simulink model "PreCNN_SAC_RL_env"  (R2025b)
settings: Solver=ode4  StartTime=0.0  StopTime=50  FixedStep=0.005  RelTol=1e-3  EnableMultiTasking=on
values from neighbouring files (symbols this model uses):
  dyn_obs = struct('p0', cell(1, num_dyn_obs), 'v', cell(1, num_dyn_obs), 'radius', cell(1, num_dyn_obs))    [genera_ostacoli_dinamici.m]    (also in visualizza_raggi_completo.m = scenario.dynamic_obstacles)
  initialGainsMultiplier = 15    [init_rl.m]    (also in report_agent.m; test.m; test_agent.m; train.m)
  logging = true    [train.m]    (also in train_agent.m; train_agent_precedente.m)
  Ts = 0.1    [init_rl.m]    (also in report_agent.m; test.m; test_agent.m; train.m)
undefined symbols (not defined in the file or in its folder): angControlTuning, angRateControlTuning, bounds, Controller, decyear, DiscIntNeverNeededParam, DroneMass, Dz, Gravity, initialConditions, Iz, leapyear, logPath_num, Nz, posControlTuning, Pz, startFlightTime, tunePositionController, UAVSampleTime, Vehicle, velControlTuning
libraries: slpidlib x14, slctrl_autotuning x8, sharedutil x4, aerolibconvert2 x3, aerolibatmos2 x2, aerolibgravity2 x2, shared6dof x2, aerolibasang x2, sensorinslib x2, deeplib x1, rllib x1, matrix_library x1
(part 4 of 5)

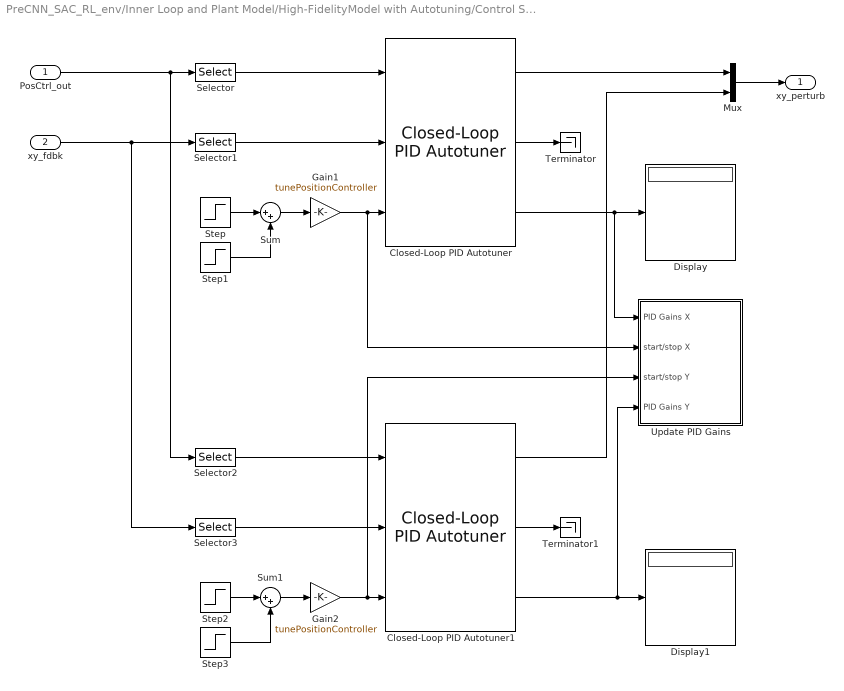
== system PreCNN_SAC_RL_env/Inner Loop and Plant Model/High-FidelityModel with Autotuning/Control System/Controller/Position Controller/Position Loop Autotuning ==
  PosCtrl_out : Inport
  xy_fdbk : Inport  Port=2
  Closed-Loop PID Autotuner : slctrl_autotuning/Closed-Loop PID Autotuner  PIDType=P  PIDForm=Parallel  TimeDomain=discrete-time  DiscreteTs=UAVSampleTime  TuningTs=0.2  UseTuningTs=off  IntegratorFormula=Forward Euler  FilterFormula=Forward Euler  ContinuousTs=0.02  Bandwidth=posControlTuning.wc  UseExternalWC=off  TargetPM=posControlTuning.pm  UseExternalPM=off  UseExternalAchievedPM=off  ExperimentMode=Superposition  PlantType=Stable  PlantSign=Positive  AmpSine=posControlTuning.sineAmp  UseExternalAmpSine=off  UseExternalFRD=off  UseExternalU0=off  UseCompanion=off  NotDeployTuningModule=off  UsePLCCoder=off  OutputMode=perturbation only  BlockDataType=single  UseExperimentGoodPort=off  UseConnectedPID=on  blockpath=[]  tunedP=0  tunedI=0  tunedD=0  tunedN=100  tunedPM=0  EstimationWindowSize=3  UseExternalTuningParams=off  SingleMultiRateVariant=SingleSamplingRate  NumEstimationPeriods=4  NumSettlingPeriods=2  NumOfPRBSPeriod=1  PRBSSignalOrder=12  ExperimentModeVariant=VariantSuperimposed  OutputChoice=VariantDonly  ConvergenceCalcVariant=ConvSuperpositionPRBSVariant
  Closed-Loop PID Autotuner1 : slctrl_autotuning/Closed-Loop PID Autotuner  PIDType=P  PIDForm=Parallel  TimeDomain=discrete-time  DiscreteTs=UAVSampleTime  TuningTs=0.2  UseTuningTs=off  IntegratorFormula=Forward Euler  FilterFormula=Forward Euler  ContinuousTs=0.02  Bandwidth=posControlTuning.wc  UseExternalWC=off  TargetPM=posControlTuning.pm  UseExternalPM=off  UseExternalAchievedPM=off  ExperimentMode=Superposition  PlantType=Stable  PlantSign=Positive  AmpSine=posControlTuning.sineAmp  UseExternalAmpSine=off  UseExternalFRD=off  UseExternalU0=off  UseCompanion=off  NotDeployTuningModule=off  UsePLCCoder=off  OutputMode=perturbation only  BlockDataType=single  UseExperimentGoodPort=off  UseConnectedPID=on  blockpath=[]  tunedP=0  tunedI=0  tunedD=0  tunedN=100  tunedPM=0  EstimationWindowSize=3  UseExternalTuningParams=off  SingleMultiRateVariant=SingleSamplingRate  NumEstimationPeriods=4  NumSettlingPeriods=2  NumOfPRBSPeriod=1  PRBSSignalOrder=12  ExperimentModeVariant=VariantSuperimposed  OutputChoice=VariantDonly  ConvergenceCalcVariant=ConvSuperpositionPRBSVariant
  Display : Display
  Display1 : Display
  Gain1 : Gain  Gain=tunePositionController
  Gain2 : Gain  Gain=tunePositionController
  Mux : Mux  Inputs=2
  Selector : Selector  InputPortWidth=2  IndexOptions=Index vector (dialog)  Indices=1  OutputSizes=1
  Selector1 : Selector  InputPortWidth=2  IndexOptions=Index vector (dialog)  Indices=1  OutputSizes=1
  Selector2 : Selector  InputPortWidth=2  IndexOptions=Index vector (dialog)  Indices=2  OutputSizes=1
  Selector3 : Selector  InputPortWidth=2  IndexOptions=Index vector (dialog)  Indices=2  OutputSizes=1
  Step : Step  Time=posControlTuning.startExpX  SampleTime=UAVSampleTime
  Step1 : Step  Time=posControlTuning.stopExpX  After=-1  SampleTime=UAVSampleTime
  Step2 : Step  Time=posControlTuning.startExpY  SampleTime=UAVSampleTime
  Step3 : Step  Time=posControlTuning.stopExpY  After=-1  SampleTime=UAVSampleTime
  Sum : Sum  Inputs=|++
  Sum1 : Sum  Inputs=|++
  Terminator : Terminator
  Terminator1 : Terminator
  Update PID Gains : Subsystem
  xy_perturb : Outport
  wires:
  PosCtrl_out/1 -> Selector2/1, Selector/1
  xy_fdbk/1 -> Selector3/1, Selector1/1
  Selector/1 -> Closed-Loop PID Autotuner/1
  Selector1/1 -> Closed-Loop PID Autotuner/2
  Sum/1 -> Gain1/1
  Step/1 -> Sum/1
  Step1/1 -> Sum/2
  Closed-Loop PID Autotuner/2 -> Terminator/1
  Mux/1 -> xy_perturb/1
  Closed-Loop PID Autotuner/1 -> Mux/1
  Selector2/1 -> Closed-Loop PID Autotuner1/1
  Selector3/1 -> Closed-Loop PID Autotuner1/2
  Step3/1 -> Sum1/2
  Step2/1 -> Sum1/1
  Sum1/1 -> Gain2/1
  Closed-Loop PID Autotuner1/2 -> Terminator1/1
  Closed-Loop PID Autotuner1/1 -> Mux/2
  Closed-Loop PID Autotuner/3 -> Update PID Gains/1(PID Gains X), Display/1
  Closed-Loop PID Autotuner1/3 -> Update PID Gains/4(PID Gains Y), Display1/1
  Gain1/1 -> Update PID Gains/2(start/stop X), Closed-Loop PID Autotuner/3
  Gain2/1 -> Update PID Gains/3(start/stop Y), Closed-Loop PID Autotuner1/3

== system PreCNN_SAC_RL_env/Inner Loop and Plant Model/High-FidelityModel with Autotuning/Control System/Controller/Position Controller/Velocity Loop Autotuning ==
  VelCtrl_out : Inport
  xxyy_fdbk : Inport  Port=2
  Closed-Loop PID Autotuner : slctrl_autotuning/Closed-Loop PID Autotuner  PIDType=PI  PIDForm=Parallel  TimeDomain=discrete-time  DiscreteTs=UAVSampleTime  TuningTs=0.2  UseTuningTs=off  IntegratorFormula=Forward Euler  FilterFormula=Forward Euler  ContinuousTs=0.02  Bandwidth=velControlTuning.wc  UseExternalWC=off  TargetPM=velControlTuning.pm  UseExternalPM=off  UseExternalAchievedPM=off  ExperimentMode=Superposition  PlantType=Stable  PlantSign=Positive  AmpSine=velControlTuning.sineAmp  UseExternalAmpSine=off  UseExternalFRD=off  UseExternalU0=off  UseCompanion=off  NotDeployTuningModule=off  UsePLCCoder=off  OutputMode=perturbation only  BlockDataType=single  UseExperimentGoodPort=off  UseConnectedPID=on  blockpath=[]  tunedP=0  tunedI=0  tunedD=0  tunedN=100  tunedPM=0  EstimationWindowSize=3  UseExternalTuningParams=off  SingleMultiRateVariant=SingleSamplingRate  NumEstimationPeriods=4  NumSettlingPeriods=2  NumOfPRBSPeriod=1  PRBSSignalOrder=12  ExperimentModeVariant=VariantSuperimposed  OutputChoice=VariantDonly  ConvergenceCalcVariant=ConvSuperpositionPRBSVariant
  Closed-Loop PID Autotuner1 : slctrl_autotuning/Closed-Loop PID Autotuner  PIDType=PI  PIDForm=Parallel  TimeDomain=discrete-time  DiscreteTs=UAVSampleTime  TuningTs=0.2  UseTuningTs=off  IntegratorFormula=Forward Euler  FilterFormula=Forward Euler  ContinuousTs=0.02  Bandwidth=velControlTuning.wc  UseExternalWC=off  TargetPM=velControlTuning.pm  UseExternalPM=off  UseExternalAchievedPM=off  ExperimentMode=Superposition  PlantType=Stable  PlantSign=Positive  AmpSine=velControlTuning.sineAmp  UseExternalAmpSine=off  UseExternalFRD=off  UseExternalU0=off  UseCompanion=off  NotDeployTuningModule=off  UsePLCCoder=off  OutputMode=perturbation only  BlockDataType=single  UseExperimentGoodPort=off  UseConnectedPID=on  blockpath=[]  tunedP=0  tunedI=0  tunedD=0  tunedN=100  tunedPM=0  EstimationWindowSize=3  UseExternalTuningParams=off  SingleMultiRateVariant=SingleSamplingRate  NumEstimationPeriods=4  NumSettlingPeriods=2  NumOfPRBSPeriod=1  PRBSSignalOrder=12  ExperimentModeVariant=VariantSuperimposed  OutputChoice=VariantDonly  ConvergenceCalcVariant=ConvSuperpositionPRBSVariant
  Display : Display
  Display1 : Display
  Gain : Gain  Gain=tunePositionController
  Gain1 : Gain  Gain=tunePositionController
  Mux : Mux  Inputs=2
  Scope : Scope
      settings: ActiveDisplayYMinimum=99.18257  ActiveDisplayYMaximum=100.62707  DataLoggingVariableName=ScopeData9
  Scope1 : Scope
      settings: DataLoggingVariableName=ScopeData10
  Selector : Selector  InputPortWidth=2  IndexOptions=Index vector (dialog)  Indices=1  OutputSizes=1
  Selector1 : Selector  InputPortWidth=2  IndexOptions=Index vector (dialog)  Indices=1  OutputSizes=1
  Selector2 : Selector  InputPortWidth=2  IndexOptions=Index vector (dialog)  Indices=2  OutputSizes=1
  Selector3 : Selector  InputPortWidth=2  IndexOptions=Index vector (dialog)  Indices=2  OutputSizes=1
  Step : Step  Time=velControlTuning.startExpX  SampleTime=UAVSampleTime
  Step1 : Step  Time=velControlTuning.stopExpX  After=-1  SampleTime=UAVSampleTime
  Step2 : Step  Time=velControlTuning.startExpY  SampleTime=UAVSampleTime
  Step3 : Step  Time=velControlTuning.stopExpY  After=-1  SampleTime=UAVSampleTime
  Sum : Sum  Inputs=|++
  Sum1 : Sum  Inputs=|++
  Update PID Gains : Subsystem
  xxyy_perturb : Outport
  wires:
  Closed-Loop PID Autotuner1/1 -> Mux/2
  Closed-Loop PID Autotuner1/2 -> Scope1/1
  Sum1/1 -> Gain1/1
  Step2/1 -> Sum1/1
  Step3/1 -> Sum1/2
  Selector3/1 -> Closed-Loop PID Autotuner1/2
  Selector2/1 -> Closed-Loop PID Autotuner1/1
  Closed-Loop PID Autotuner/1 -> Mux/1
  Mux/1 -> xxyy_perturb/1
  Closed-Loop PID Autotuner/2 -> Scope/1
  Step1/1 -> Sum/2
  Step/1 -> Sum/1
  Sum/1 -> Gain/1
  Selector1/1 -> Closed-Loop PID Autotuner/2
  Selector/1 -> Closed-Loop PID Autotuner/1
  xxyy_fdbk/1 -> Selector1/1, Selector3/1
  VelCtrl_out/1 -> Selector/1, Selector2/1
  Closed-Loop PID Autotuner/3 -> Update PID Gains/1(PID Gains XX), Display/1
  Closed-Loop PID Autotuner1/3 -> Update PID Gains/4(PID Gains YY), Display1/1
  Gain/1 -> Update PID Gains/2(start/stop XX), Closed-Loop PID Autotuner/3
  Gain1/1 -> Update PID Gains/3(start/stop YY), Closed-Loop PID Autotuner1/3

== system PreCNN_SAC_RL_env/Inner Loop and Plant Model/High-FidelityModel with Autotuning/Plant Model/AC model/Drag Calculation/Drag Calc ==
  Density : Inport  Unit=kg/m^3
  vel : Inport  Port=2  Unit=m/s
  Dynamic Pressure : aerolibasang/Dynamic Pressure
  Gain : Gain  Gain=[.25 .25]
  Mux1 : Mux  Inputs=2
  Product : Product  Inputs=3  RndMeth=Zero
  diameter : Constant  Value=Vehicle.Airframe.diameter  SampleTime=0
  dragCoeff : Constant  Value=Vehicle.Airframe.Cdx  SampleTime=0
  drag : Outport  Unit=N  VectorParamsAs1DForOutWhenUnconnected=off
  wires:
  Product/1 -> drag/1
  dragCoeff/1 -> Product/3  "Cd"
  Dynamic Pressure/1 -> Product/1  "q"
  diameter/1 -> Gain/1, Mux1/2
  Mux1/1 -> Product/2  "S"
  Gain/1 -> Mux1/1
  vel/1 -> Dynamic Pressure/1
  Density/1 -> Dynamic Pressure/2

== system PreCNN_SAC_RL_env/Inner Loop and Plant Model/High-FidelityModel with Autotuning/Plant Model/AC model/Motor Forces and Torques/For Each Subsystem ==
  Vb : Inport  PortDimensions=3
  rho : Inport  Port=2  PortDimensions=1
  Omega : Inport  Port=3
  w : Inport  Port=4  Partition=on  PartitionDimension=2  PartitionWidth=1  PartitionOffset=0
  D : Inport  Port=5  Partition=on  PartitionDimension=2  PartitionWidth=1  PartitionOffset=0
  For Each : ForEach  DisableCoverage=on
  RotorDynamics : Subsystem  TreatAsAtomicUnit=on
      mask init:
      | aeroicon('aeroblk');
      settings: RTWFcnNameOpts=Use subsystem name  RTWFileNameOpts=Use function name
  Forces : Outport  ConcatenationDimension=2  VectorParamsAs1DForOutWhenUnconnected=off
  Moments : Outport  Port=2  ConcatenationDimension=2  VectorParamsAs1DForOutWhenUnconnected=off
  wires:
  RotorDynamics/1(Fxyz) -> Forces/1
  RotorDynamics/2(Mxyz) -> Moments/1
  Vb/1 -> RotorDynamics/1(Vb)
  Omega/1 -> RotorDynamics/2(pqr)
  rho/1 -> RotorDynamics/3(rho)
  D/1 -> RotorDynamics/5(Arm)
  w/1 -> RotorDynamics/4(w)

== system PreCNN_SAC_RL_env/Inner Loop and Plant Model/High-FidelityModel with Autotuning/Plant Model/AC model/Motor Forces and Torques/MotorsToW ==
  motors_datin : Inport
  Motordirections : Gain  Gain=[1 -1 1 -1]  ParamDataTypeStr=single  OutDataTypeStr=Inherit: Inherit via back propagation  SaturateOnIntegerOverflow=on
  Motordirections1 : Gain  Gain=[1 -1 1 -1]  ParamDataTypeStr=single  OutDataTypeStr=Inherit: Inherit via back propagation  SaturateOnIntegerOverflow=on
  Saturation5 : Saturate  UpperLimit=Vehicle.Motor.maxLimit  LowerLimit=Vehicle.Motor.minLimit  OutDataTypeStr=Inherit: Inherit via back propagation
  Signed Sqrt : Sqrt  Operator=signedSqrt  OutDataTypeStr=Inherit: Inherit via back propagation
  motorsToW2_Gain : Gain  Gain=Vehicle.Motor.commandToW2Gain  ParamDataTypeStr=single  OutDataTypeStr=Inherit: Inherit via back propagation  SaturateOnIntegerOverflow=on
  omegas_datout : Outport  VectorParamsAs1DForOutWhenUnconnected=off
  wires:
  motorsToW2_Gain/1 -> Signed Sqrt/1
  Motordirections/1 -> Saturation5/1
  Saturation5/1 -> Motordirections1/1
  Motordirections1/1 -> motorsToW2_Gain/1
  Signed Sqrt/1 -> omegas_datout/1
  motors_datin/1 -> Motordirections/1

== system PreCNN_SAC_RL_env/Inner Loop and Plant Model/High-FidelityModel with Autotuning/Plant Model/Bus setup/Generate GPS Data/Scale and Assemble GPS Data  ==
  Xe : Inport
  Ve : Inport  Port=2
  Angle Conversion1 : aerolibconvert2/Angle Conversion  IU=rad  OU=deg
  Bus Creator1 : BusCreator  Inputs=9  OutDataTypeStr=Bus: gps_raw_int  NonVirtualBus=on
      settings: InheritFromInputs=off
  Clock : Clock
      settings: AttributesFormatString=Decimation: %<Decimation>
  Data Type Conversion : DataTypeConversion  OutDataTypeStr=uint32  SaturateOnIntegerOverflow=off  RndMeth=Floor
  Demux1 : Demux  Outputs=3
  Demux2 : Demux  Outputs=2
  Embedded MATLAB Function1 : MATLAB Function  TreatAsAtomicUnit=on
  Fcn : Fcn  Expr=sqrt(u(1)^2+u(2)^2+u(3)^2)
  Flat Earth to LLA : FlatEarth2LLA  R=6378137  LL0=uavIC_latLon
  Gain : Gain  Gain=1e7  OutDataTypeStr=int32
  Gain1 : Gain  Gain=1e7  OutDataTypeStr=int32
  Gain2 : Gain  Gain=-1e3  OutDataTypeStr=int32
  Gain3 : Gain  Gain=1e2  OutDataTypeStr=uint16
  Gain4 : Gain  Gain=1e2  OutDataTypeStr=uint16
  Rate Transition1 : RateTransition  Commented=through  OutPortSampleTime=0.005
  Terminator : Terminator
  Zero level trust : Constant  Value=0
      settings: AttributesFormatString=%<Value>
  Zero level trust5 : Constant  Value=3  OutDataTypeStr=uint8
      settings: AttributesFormatString=%<Value>
  Zero level trust6 : Constant  Value=80  OutDataTypeStr=uint16
      settings: AttributesFormatString=%<Value>
  Zero level trust7 : Constant  Value=80  OutDataTypeStr=uint16
      settings: AttributesFormatString=%<Value>
  Out1 : Outport
  wires:
  Demux2/1 -> Gain/1
  Gain/1 -> Bus Creator1/3
  Gain4/1 -> Bus Creator1/9
  Demux2/2 -> Gain1/1
  Embedded MATLAB Function1/1(cog) -> Angle Conversion1/1
  Rate Transition1/1 -> Bus Creator1/1
  Zero level trust6/1 -> Bus Creator1/6
  Gain3/1 -> Bus Creator1/8
  Clock/1 -> Data Type Conversion/1
  Ve/1 -> Demux1/1, Fcn/1
  Zero level trust7/1 -> Bus Creator1/7
  Data Type Conversion/1 -> Rate Transition1/1
  Demux1/2 -> Embedded MATLAB Function1/2(Ve)
  Zero level trust5/1 -> Bus Creator1/2
  Demux1/1 -> Embedded MATLAB Function1/1(Vn)
  Flat Earth to LLA/1 -> Demux2/1  "gps_latLon"
  Gain2/1 -> Bus Creator1/5
  Fcn/1 -> Gain3/1  "gps_sog"
  Gain1/1 -> Bus Creator1/4
  Flat Earth to LLA/2 -> Gain2/1  "gps_h"
  Zero level trust/1 -> Flat Earth to LLA/2
  Angle Conversion1/1 -> Gain4/1  "gps_cog"
  Demux1/3 -> Terminator/1
  Xe/1 -> Flat Earth to LLA/1
  Bus Creator1/1 -> Out1/1

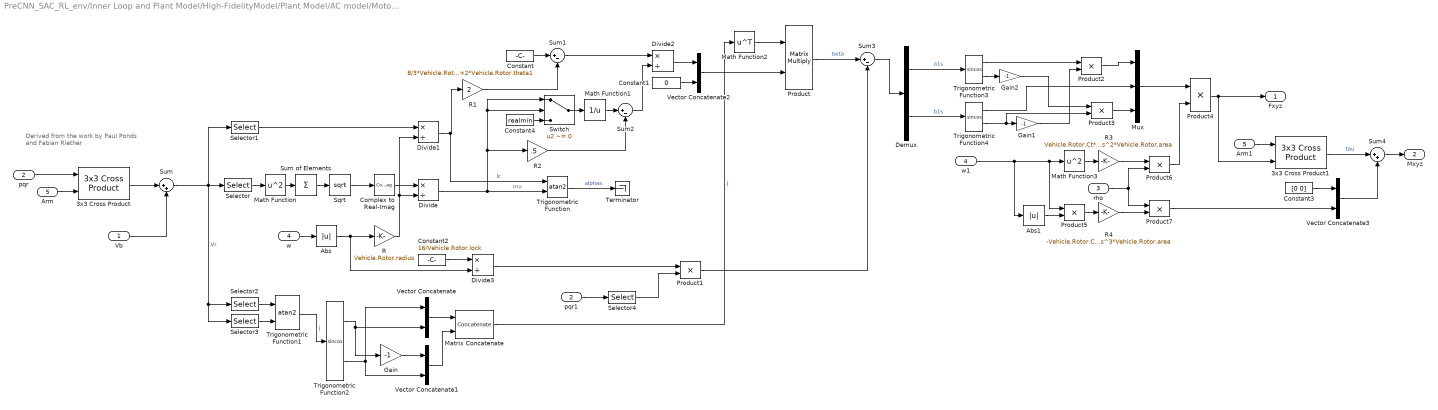
== system PreCNN_SAC_RL_env/Inner Loop and Plant Model/High-FidelityModel/Plant Model/AC model/Motor Forces and Torques/For Each Subsystem/RotorDynamics ==
  note: Derived from the work by Paul Ponds
      | and Fabian Riether
  Vb : Inport  PortDimensions=3
  pqr : Inport  Port=2  PortDimensions=3
  rho : Inport  Port=3  PortDimensions=1
  w : Inport  Port=4  PortDimensions=[1 1]
  Arm : Inport  Port=5  PortDimensions=[3 1]
  3x3 Cross Product : sharedutil/3x3 Cross Product  aMode=aMode
  3x3 Cross Product1 : sharedutil/3x3 Cross Product  aMode=aMode
  Abs : Abs  SaturateOnIntegerOverflow=off
  Abs1 : Abs  SaturateOnIntegerOverflow=off
  Arm1 : InportShadow  Port=5  PortDimensions=[3 1]
  Complex to Real-Imag : ComplexToRealImag  Output=Real
  Constant : Constant  Value=8/3*Vehicle.Rotor.theta0+2*Vehicle.Rotor.theta1
  Constant1 : Constant  Value=0
  Constant2 : Constant  Value=16/Vehicle.Rotor.lock
  Constant3 : Constant  Value=[0 0]
  Constant4 : Constant  Value=realmin
  Demux : Demux  Outputs=2
  Divide{,1..3} (4 alike) : Product  Inputs=*/
  Gain : Gain  Gain=-1
  Gain1 : Gain  Gain=-1
  Gain2 : Gain  Gain=-1
  Math Function : Math  Operator=square  SignedPower=on
  Math Function1 : Math  Operator=reciprocal  SignedPower=on
  Math Function2 : Math  Operator=transpose  SignedPower=on
  Math Function3 : Math  Operator=square  SignedPower=on
  Matrix Concatenate : Concatenate  Mode=Multidimensional array  ConcatenateDimension=2
  Mux : Mux  Inputs=3
  Product : Product  Multiplication=Matrix(*)
  Product{1..7} (7 alike) : Product
  R : Gain  Gain=Vehicle.Rotor.radius
  R1 : Gain  Gain=2
  R2 : Gain  Gain=.5
  R3 : Gain  Gain=Vehicle.Rotor.Ct*Vehicle.Rotor.radius^2*Vehicle.Rotor.area
  R4 : Gain  Gain=-Vehicle.Rotor.Cq*Vehicle.Rotor.radius^3*Vehicle.Rotor.area
  Selector : Selector  InputPortWidth=3  IndexOptions=Index vector (dialog)  Indices=[1 2]  OutputSizes=1
  Selector1 : Selector  InputPortWidth=3  IndexOptions=Index vector (dialog)  Indices=[3]  OutputSizes=1
  Selector2 : Selector  InputPortWidth=3  IndexOptions=Index vector (dialog)  Indices=[2]  OutputSizes=1
  Selector3 : Selector  InputPortWidth=3  IndexOptions=Index vector (dialog)  Indices=[1]  OutputSizes=1
  Selector4 : Selector  InputPortWidth=3  IndexOptions=Index vector (dialog)  Indices=[2 1]  OutputSizes=1
  Sqrt : Sqrt  OutputSignalType=complex
  Sum : Sum  Inputs=|++
  Sum of Elements : Sum  Inputs=+
  Sum1 : Sum  Inputs=|+-
  Sum2 : Sum  Inputs=|+-
  Sum3 : Sum  Inputs=|+-
  Sum4 : Sum  Inputs=|++
  Switch : Switch  Criteria=u2 ~= 0  SaturateOnIntegerOverflow=off  InputSameDT=off
  Terminator : Terminator
  Trigonometric Function : Trigonometry  Operator=atan2
  Trigonometric Function1 : Trigonometry  Operator=atan2
  Trigonometric Function2 : Trigonometry  Operator=sincos
  Trigonometric Function3 : Trigonometry  Operator=sincos
  Trigonometric Function4 : Trigonometry  Operator=sincos
  Vector Concatenate{,1..3} (4 alike) : Concatenate
  pqr1 : InportShadow  Port=2  PortDimensions=3
  w1 : InportShadow  Port=4  PortDimensions=[1 1]
  Fxyz : Outport  PortDimensions=[3 1]  VectorParamsAs1DForOutWhenUnconnected=off
  Mxyz : Outport  Port=2  PortDimensions=[3 1]  VectorParamsAs1DForOutWhenUnconnected=off
  wires:
  Complex to Real-Imag/1 -> Divide/1
  Sqrt/1 -> Complex to Real-Imag/1
  Constant4/1 -> Switch/3
  Switch/1 -> Math Function1/1
  Product1/1 -> Sum3/2
  rho/1 -> Product7/1, Product6/2
  Product7/1 -> Vector Concatenate3/2
  Product6/1 -> Product4/2
  Sum4/1 -> Mxyz/1
  3x3 Cross Product1/1 -> Sum4/1  "tau"
  Product4/1 -> Fxyz/1, 3x3 Cross Product1/2
  Arm1/1 -> 3x3 Cross Product1/1
  Vector Concatenate3/1 -> Sum4/2
  Constant3/1 -> Vector Concatenate3/1
  R4/1 -> Product7/2
  Product5/1 -> R4/1
  Abs1/1 -> Product5/2
  R3/1 -> Product6/1
  Mux/1 -> Product4/1
  Gain2/1 -> Product3/1
  Product3/1 -> Mux/3
  Trigonometric Function3/2 -> Gain2/1
  Trigonometric Function4/1 -> Mux/2
  Product2/1 -> Mux/1
  Trigonometric Function3/1 -> Product2/1
  Gain1/1 -> Product2/2
  Trigonometric Function4/2 -> Gain1/1, Product3/2
  Demux/2 -> Trigonometric Function4/1  "b1s"
  Demux/1 -> Trigonometric Function3/1  "a1s"
  Sum3/1 -> Demux/1
  Math Function3/1 -> R3/1
  w1/1 -> Math Function3/1, Product5/1, Abs1/1
  Divide3/1 -> Product1/1
  Abs/1 -> R/1, Divide3/2
  Selector4/1 -> Product1/2
  pqr1/1 -> Selector4/1
  Constant2/1 -> Divide3/1
  Product/1 -> Sum3/1  "beta"
  Math Function2/1 -> Product/1
  Vector Concatenate2/1 -> Product/2
  Constant1/1 -> Vector Concatenate2/2
  Divide2/1 -> Vector Concatenate2/1
  Sum2/1 -> Divide2/2
  R2/1 -> Sum2/2
  Math Function1/1 -> Sum2/1
  Sum1/1 -> Divide2/1
  R1/1 -> Sum1/2
  Constant/1 -> Sum1/1
  Matrix Concatenate/1 -> Math Function2/1  "J"
  Vector Concatenate1/1 -> Matrix Concatenate/2
  Vector Concatenate/1 -> Matrix Concatenate/1
  Trigonometric Function2/1 -> Gain/1, Vector Concatenate/2
  Gain/1 -> Vector Concatenate1/1
  Trigonometric Function2/2 -> Vector Concatenate/1, Vector Concatenate1/2
  Trigonometric Function1/1 -> Trigonometric Function2/1  "j"
  Selector3/1 -> Trigonometric Function1/2
  Selector2/1 -> Trigonometric Function1/1
  Trigonometric Function/1 -> Terminator/1  "alphas"
  Divide1/1 -> Trigonometric Function/1, R1/1  "lc"
  Selector1/1 -> Divide1/1
  Divide/1 -> Trigonometric Function/2, Switch/1, Switch/2, R2/1  "mu"
  R/1 -> Divide/2, Divide1/2
  w/1 -> Abs/1
  Arm/1 -> 3x3 Cross Product/2
  pqr/1 -> 3x3 Cross Product/1
  Sum of Elements/1 -> Sqrt/1
  Math Function/1 -> Sum of Elements/1
  Selector/1 -> Math Function/1
  Sum/1 -> Selector/1, Selector1/1, Selector2/1, Selector3/1  "Vr"
  Vb/1 -> Sum/2
  3x3 Cross Product/1 -> Sum/1

== system PreCNN_SAC_RL_env/Inner Loop and Plant Model/High-FidelityModel with Autotuning/Control System/Controller/Attitude Controller/Angle Loop Autotuning/Update PID Gains ==
  PID Gains pitch : Inport
  start/stop pitch : Inport  Port=2
  start/stop roll : Inport  Port=3
  PID Gains roll : Inport  Port=4
  Unit Delay1 : UnitDelay  SampleTime=UAVSampleTime  HasFrameUpgradeWarning=on
  Unit Delay2 : UnitDelay  SampleTime=UAVSampleTime  HasFrameUpgradeWarning=on
  Update PID Gains pitch : Subsystem
  Update PID Gains roll : Subsystem
  wires:
  PID Gains roll/1 -> Update PID Gains roll/1(PID Gains Roll)
  PID Gains pitch/1 -> Update PID Gains pitch/1(PID Gains pitch)
  Unit Delay2/1 -> Update PID Gains pitch/Trigger
  Unit Delay1/1 -> Update PID Gains roll/Trigger
  start/stop pitch/1 -> Unit Delay2/1
  start/stop roll/1 -> Unit Delay1/1

== system PreCNN_SAC_RL_env/Inner Loop and Plant Model/High-FidelityModel with Autotuning/Control System/Controller/Attitude Controller/Angular Velocity Loop Autotuning/Update PID Gains ==
  PID Gains pitchrate : Inport
  start/stop pitchrate : Inport  Port=2
  start/stop rollrate : Inport  Port=3
  PID Gains rollrate : Inport  Port=4
  Unit Delay1 : UnitDelay  SampleTime=UAVSampleTime  HasFrameUpgradeWarning=on
  Unit Delay2 : UnitDelay  SampleTime=UAVSampleTime  HasFrameUpgradeWarning=on
  Update PID Gains pitchrate : Subsystem
  Update PID Gains rollrate : Subsystem
  wires:
  PID Gains rollrate/1 -> Update PID Gains rollrate/1(PID Gains rollrate)
  PID Gains pitchrate/1 -> Update PID Gains pitchrate/1(PID Gains pitchrate)
  Unit Delay2/1 -> Update PID Gains pitchrate/Trigger
  Unit Delay1/1 -> Update PID Gains rollrate/Trigger
  start/stop rollrate/1 -> Unit Delay1/1
  start/stop pitchrate/1 -> Unit Delay2/1

== system PreCNN_SAC_RL_env/Inner Loop and Plant Model/High-FidelityModel with Autotuning/Control System/Controller/Position Controller/Position Loop Autotuning/Update PID Gains ==
  PID Gains X : Inport
  start/stop X : Inport  Port=2
  start/stop Y : Inport  Port=3
  PID Gains Y : Inport  Port=4
  Unit Delay1 : UnitDelay  SampleTime=UAVSampleTime  HasFrameUpgradeWarning=on
  Unit Delay2 : UnitDelay  SampleTime=UAVSampleTime  HasFrameUpgradeWarning=on
  Update PID Gains X : Subsystem
  Update PID Gains Y : Subsystem
  wires:
  PID Gains Y/1 -> Update PID Gains Y/1(PID Gains Y)
  PID Gains X/1 -> Update PID Gains X/1(PID Gains X)
  Unit Delay2/1 -> Update PID Gains X/Trigger
  Unit Delay1/1 -> Update PID Gains Y/Trigger
  start/stop X/1 -> Unit Delay2/1
  start/stop Y/1 -> Unit Delay1/1

== system PreCNN_SAC_RL_env/Inner Loop and Plant Model/High-FidelityModel with Autotuning/Control System/Controller/Position Controller/Velocity Loop Autotuning/Update PID Gains ==
  PID Gains XX : Inport
  start/stop XX : Inport  Port=2
  start/stop YY : Inport  Port=3
  PID Gains YY : Inport  Port=4
  Unit Delay1 : UnitDelay  SampleTime=UAVSampleTime  HasFrameUpgradeWarning=on
  Unit Delay2 : UnitDelay  SampleTime=UAVSampleTime  HasFrameUpgradeWarning=on
  Update PID Gains XX : Subsystem
  Update PID Gains YY : Subsystem
  wires:
  PID Gains YY/1 -> Update PID Gains YY/1(PID Gains YY)
  PID Gains XX/1 -> Update PID Gains XX/1(PID Gains XX)
  Unit Delay2/1 -> Update PID Gains XX/Trigger
  Unit Delay1/1 -> Update PID Gains YY/Trigger
  start/stop XX/1 -> Unit Delay2/1
  start/stop YY/1 -> Unit Delay1/1

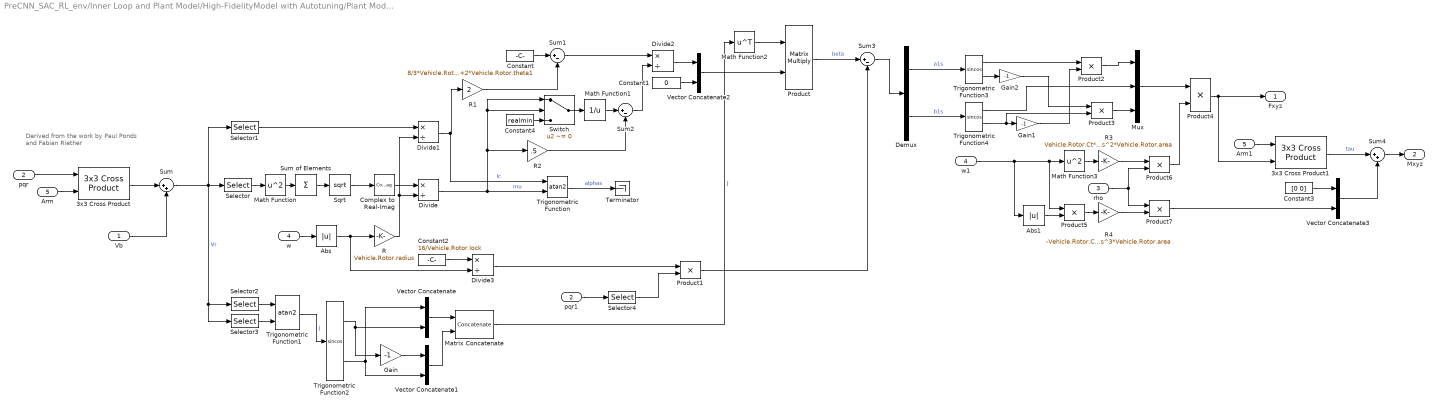
== system PreCNN_SAC_RL_env/Inner Loop and Plant Model/High-FidelityModel with Autotuning/Plant Model/AC model/Motor Forces and Torques/For Each Subsystem/RotorDynamics ==
  note: Derived from the work by Paul Ponds
      | and Fabian Riether
  Vb : Inport  PortDimensions=3
  pqr : Inport  Port=2  PortDimensions=3
  rho : Inport  Port=3  PortDimensions=1
  w : Inport  Port=4  PortDimensions=[1 1]
  Arm : Inport  Port=5  PortDimensions=[3 1]
  3x3 Cross Product : sharedutil/3x3 Cross Product  aMode=aMode
  3x3 Cross Product1 : sharedutil/3x3 Cross Product  aMode=aMode
  Abs : Abs  SaturateOnIntegerOverflow=off
  Abs1 : Abs  SaturateOnIntegerOverflow=off
  Arm1 : InportShadow  Port=5  PortDimensions=[3 1]
  Complex to Real-Imag : ComplexToRealImag  Output=Real
  Constant : Constant  Value=8/3*Vehicle.Rotor.theta0+2*Vehicle.Rotor.theta1
  Constant1 : Constant  Value=0
  Constant2 : Constant  Value=16/Vehicle.Rotor.lock
  Constant3 : Constant  Value=[0 0]
  Constant4 : Constant  Value=realmin
  Demux : Demux  Outputs=2
  Divide{,1..3} (4 alike) : Product  Inputs=*/
  Gain : Gain  Gain=-1
  Gain1 : Gain  Gain=-1
  Gain2 : Gain  Gain=-1
  Math Function : Math  Operator=square  SignedPower=on
  Math Function1 : Math  Operator=reciprocal  SignedPower=on
  Math Function2 : Math  Operator=transpose  SignedPower=on
  Math Function3 : Math  Operator=square  SignedPower=on
  Matrix Concatenate : Concatenate  Mode=Multidimensional array  ConcatenateDimension=2
  Mux : Mux  Inputs=3
  Product : Product  Multiplication=Matrix(*)
  Product{1..7} (7 alike) : Product
  R : Gain  Gain=Vehicle.Rotor.radius
  R1 : Gain  Gain=2
  R2 : Gain  Gain=.5
  R3 : Gain  Gain=Vehicle.Rotor.Ct*Vehicle.Rotor.radius^2*Vehicle.Rotor.area
  R4 : Gain  Gain=-Vehicle.Rotor.Cq*Vehicle.Rotor.radius^3*Vehicle.Rotor.area
  Selector : Selector  InputPortWidth=3  IndexOptions=Index vector (dialog)  Indices=[1 2]  OutputSizes=1
  Selector1 : Selector  InputPortWidth=3  IndexOptions=Index vector (dialog)  Indices=[3]  OutputSizes=1
  Selector2 : Selector  InputPortWidth=3  IndexOptions=Index vector (dialog)  Indices=[2]  OutputSizes=1
  Selector3 : Selector  InputPortWidth=3  IndexOptions=Index vector (dialog)  Indices=[1]  OutputSizes=1
  Selector4 : Selector  InputPortWidth=3  IndexOptions=Index vector (dialog)  Indices=[2 1]  OutputSizes=1
  Sqrt : Sqrt  OutputSignalType=complex
  Sum : Sum  Inputs=|++
  Sum of Elements : Sum  Inputs=+
  Sum1 : Sum  Inputs=|+-
  Sum2 : Sum  Inputs=|+-
  Sum3 : Sum  Inputs=|+-
  Sum4 : Sum  Inputs=|++
  Switch : Switch  Criteria=u2 ~= 0  SaturateOnIntegerOverflow=off  InputSameDT=off
  Terminator : Terminator
  Trigonometric Function : Trigonometry  Operator=atan2
  Trigonometric Function1 : Trigonometry  Operator=atan2
  Trigonometric Function2 : Trigonometry  Operator=sincos
  Trigonometric Function3 : Trigonometry  Operator=sincos
  Trigonometric Function4 : Trigonometry  Operator=sincos
  Vector Concatenate{,1..3} (4 alike) : Concatenate
  pqr1 : InportShadow  Port=2  PortDimensions=3
  w1 : InportShadow  Port=4  PortDimensions=[1 1]
  Fxyz : Outport  PortDimensions=[3 1]  VectorParamsAs1DForOutWhenUnconnected=off
  Mxyz : Outport  Port=2  PortDimensions=[3 1]  VectorParamsAs1DForOutWhenUnconnected=off
  wires:
  Complex to Real-Imag/1 -> Divide/1
  Sqrt/1 -> Complex to Real-Imag/1
  Constant4/1 -> Switch/3
  Switch/1 -> Math Function1/1
  Product1/1 -> Sum3/2
  rho/1 -> Product7/1, Product6/2
  Product7/1 -> Vector Concatenate3/2
  Product6/1 -> Product4/2
  Sum4/1 -> Mxyz/1
  3x3 Cross Product1/1 -> Sum4/1  "tau"
  Product4/1 -> Fxyz/1, 3x3 Cross Product1/2
  Arm1/1 -> 3x3 Cross Product1/1
  Vector Concatenate3/1 -> Sum4/2
  Constant3/1 -> Vector Concatenate3/1
  R4/1 -> Product7/2
  Product5/1 -> R4/1
  Abs1/1 -> Product5/2
  R3/1 -> Product6/1
  Mux/1 -> Product4/1
  Gain2/1 -> Product3/1
  Product3/1 -> Mux/3
  Trigonometric Function3/2 -> Gain2/1
  Trigonometric Function4/1 -> Mux/2
  Product2/1 -> Mux/1
  Trigonometric Function3/1 -> Product2/1
  Gain1/1 -> Product2/2
  Trigonometric Function4/2 -> Gain1/1, Product3/2
  Demux/2 -> Trigonometric Function4/1  "b1s"
  Demux/1 -> Trigonometric Function3/1  "a1s"
  Sum3/1 -> Demux/1
  Math Function3/1 -> R3/1
  w1/1 -> Math Function3/1, Product5/1, Abs1/1
  Divide3/1 -> Product1/1
  Abs/1 -> R/1, Divide3/2
  Selector4/1 -> Product1/2
  pqr1/1 -> Selector4/1
  Constant2/1 -> Divide3/1
  Product/1 -> Sum3/1  "beta"
  Math Function2/1 -> Product/1
  Vector Concatenate2/1 -> Product/2
  Constant1/1 -> Vector Concatenate2/2
  Divide2/1 -> Vector Concatenate2/1
  Sum2/1 -> Divide2/2
  R2/1 -> Sum2/2
  Math Function1/1 -> Sum2/1
  Sum1/1 -> Divide2/1
  R1/1 -> Sum1/2
  Constant/1 -> Sum1/1
  Matrix Concatenate/1 -> Math Function2/1  "J"
  Vector Concatenate1/1 -> Matrix Concatenate/2
  Vector Concatenate/1 -> Matrix Concatenate/1
  Trigonometric Function2/1 -> Gain/1, Vector Concatenate/2
  Gain/1 -> Vector Concatenate1/1
  Trigonometric Function2/2 -> Vector Concatenate/1, Vector Concatenate1/2
  Trigonometric Function1/1 -> Trigonometric Function2/1  "j"
  Selector3/1 -> Trigonometric Function1/2
  Selector2/1 -> Trigonometric Function1/1
  Trigonometric Function/1 -> Terminator/1  "alphas"
  Divide1/1 -> Trigonometric Function/1, R1/1  "lc"
  Selector1/1 -> Divide1/1
  Divide/1 -> Trigonometric Function/2, Switch/1, Switch/2, R2/1  "mu"
  R/1 -> Divide/2, Divide1/2
  w/1 -> Abs/1
  Arm/1 -> 3x3 Cross Product/2
  pqr/1 -> 3x3 Cross Product/1
  Sum of Elements/1 -> Sqrt/1
  Math Function/1 -> Sum of Elements/1
  Selector/1 -> Math Function/1
  Sum/1 -> Selector/1, Selector1/1, Selector2/1, Selector3/1  "Vr"
  Vb/1 -> Sum/2
  3x3 Cross Product/1 -> Sum/1

== system PreCNN_SAC_RL_env/Inner Loop and Plant Model/High-FidelityModel with Autotuning/Control System/Controller/Attitude Controller/Angle Loop Autotuning/Update PID Gains/Update PID Gains pitch ==
  PID Gains pitch : Inport
  Trigger : TriggerPort  TriggerType=falling  VariantControl=Variant  PortDimensions=1
  Bus Selector : BusSelector  OutputSignals=P
  Write PID Gains : DataStoreWrite  DataStoreName=AttitudeLoopGainsPitch  IndexOptions=Index vector (dialog)  Indices=1  OutputSizes=1
  wires:
  PID Gains pitch/1 -> Bus Selector/1
  Bus Selector/1 -> Write PID Gains/1  "<P>"

== system PreCNN_SAC_RL_env/Inner Loop and Plant Model/High-FidelityModel with Autotuning/Control System/Controller/Attitude Controller/Angle Loop Autotuning/Update PID Gains/Update PID Gains roll ==
  PID Gains Roll : Inport
  Trigger : TriggerPort  TriggerType=falling  VariantControl=Variant  PortDimensions=1
  Bus Selector : BusSelector  OutputSignals=P
  Write PID Gains : DataStoreWrite  DataStoreName=AttitudeLoopGainsRoll  IndexOptions=Index vector (dialog)  Indices=1  OutputSizes=1
  wires:
  PID Gains Roll/1 -> Bus Selector/1
  Bus Selector/1 -> Write PID Gains/1  "<P>"

== system PreCNN_SAC_RL_env/Inner Loop and Plant Model/High-FidelityModel with Autotuning/Control System/Controller/Attitude Controller/Angular Velocity Loop Autotuning/Update PID Gains/Update PID Gains pitchrate ==
  PID Gains pitchrate : Inport
  Trigger : TriggerPort  TriggerType=falling  VariantControl=Variant  PortDimensions=1
  Bus Selector : BusSelector  OutputSignals=P,I,D,N
  Mux : Mux
  Write PID Gains : DataStoreWrite  DataStoreName=AttitudeLoopGainsPitchRate  IndexOptions=Index vector (dialog)  Indices=1  OutputSizes=1
  wires:
  Mux/1 -> Write PID Gains/1
  PID Gains pitchrate/1 -> Bus Selector/1
  Bus Selector/1 -> Mux/1  "<P>"
  Bus Selector/2 -> Mux/2  "<I>"
  Bus Selector/3 -> Mux/3  "<D>"
  Bus Selector/4 -> Mux/4  "<N>"

== system PreCNN_SAC_RL_env/Inner Loop and Plant Model/High-FidelityModel with Autotuning/Control System/Controller/Attitude Controller/Angular Velocity Loop Autotuning/Update PID Gains/Update PID Gains rollrate ==
  PID Gains rollrate : Inport
  Trigger : TriggerPort  TriggerType=falling  VariantControl=Variant  PortDimensions=1
  Bus Selector : BusSelector  OutputSignals=P,I,D,N
  Mux : Mux
  Write PID Gains : DataStoreWrite  DataStoreName=AttitudeLoopGainsRollRate  IndexOptions=Index vector (dialog)  Indices=1  OutputSizes=1
  wires:
  Mux/1 -> Write PID Gains/1
  PID Gains rollrate/1 -> Bus Selector/1
  Bus Selector/1 -> Mux/1  "<P>"
  Bus Selector/2 -> Mux/2  "<I>"
  Bus Selector/3 -> Mux/3  "<D>"
  Bus Selector/4 -> Mux/4  "<N>"

== system PreCNN_SAC_RL_env/Inner Loop and Plant Model/High-FidelityModel with Autotuning/Control System/Controller/Position Controller/Position Loop Autotuning/Update PID Gains/Update PID Gains X ==
  PID Gains X : Inport
  Trigger : TriggerPort  TriggerType=falling  VariantControl=Variant  PortDimensions=1
  Bus Selector : BusSelector  OutputSignals=P
  Write PID Gains : DataStoreWrite  DataStoreName=PosLoopGainsX  IndexOptions=Index vector (dialog)  Indices=1  OutputSizes=1
  wires:
  PID Gains X/1 -> Bus Selector/1
  Bus Selector/1 -> Write PID Gains/1  "<P>"

== system PreCNN_SAC_RL_env/Inner Loop and Plant Model/High-FidelityModel with Autotuning/Control System/Controller/Position Controller/Position Loop Autotuning/Update PID Gains/Update PID Gains Y ==
  PID Gains Y : Inport
  Trigger : TriggerPort  TriggerType=falling  VariantControl=Variant  PortDimensions=1
  Bus Selector : BusSelector  OutputSignals=P
  Write PID Gains : DataStoreWrite  DataStoreName=PosLoopGainsY  IndexOptions=Index vector (dialog)  Indices=1  OutputSizes=1
  wires:
  PID Gains Y/1 -> Bus Selector/1
  Bus Selector/1 -> Write PID Gains/1  "<P>"

== system PreCNN_SAC_RL_env/Inner Loop and Plant Model/High-FidelityModel with Autotuning/Control System/Controller/Position Controller/Velocity Loop Autotuning/Update PID Gains/Update PID Gains XX ==
  PID Gains XX : Inport
  Trigger : TriggerPort  TriggerType=falling  VariantControl=Variant  PortDimensions=1
  Bus Selector : BusSelector  OutputSignals=P,I
  Mux : Mux  Inputs=2
  Write PID Gains : DataStoreWrite  DataStoreName=PosLoopGainsXX  IndexOptions=Index vector (dialog)  Indices=1  OutputSizes=1
  wires:
  Mux/1 -> Write PID Gains/1
  Bus Selector/2 -> Mux/2  "<I>"
  Bus Selector/1 -> Mux/1  "<P>"
  PID Gains XX/1 -> Bus Selector/1

== system PreCNN_SAC_RL_env/Inner Loop and Plant Model/High-FidelityModel with Autotuning/Control System/Controller/Position Controller/Velocity Loop Autotuning/Update PID Gains/Update PID Gains YY ==
  PID Gains YY : Inport
  Trigger : TriggerPort  TriggerType=falling  VariantControl=Variant  PortDimensions=1
  Bus Selector : BusSelector  OutputSignals=P,I
  Mux : Mux  Inputs=2
  Write PID Gains : DataStoreWrite  DataStoreName=PosLoopGainsYY  IndexOptions=Index vector (dialog)  Indices=1  OutputSizes=1
  wires:
  Mux/1 -> Write PID Gains/1
  Bus Selector/2 -> Mux/2  "<I>"
  Bus Selector/1 -> Mux/1  "<P>"
  PID Gains YY/1 -> Bus Selector/1

== matlab function PreCNN_SAC_RL_env/Inner Loop and Plant Model/High-FidelityModel with Autotuning/Control System/Controller/Yaw Controller/MATLAB Function ==
  data: u input; y output
function y = wrapYaw(u)
%u error in rad in -2pi to 2pi

if (u>pi)
    y = u-2*pi;
elseif(u<-pi)
    y = u +2*pi;
else
    y=u;
end

== matlab function PreCNN_SAC_RL_env/Inner Loop and Plant Model/High-FidelityModel with Autotuning/Control System/Controller/Yaw Controller/MATLAB Function1 ==
  data: u input; y output
function y = wrapYaw(u)
%u error in rad in -2pi to 2pi

if (u>pi)
    y = u-2*pi;
elseif(u<-pi)
    y = u +2*pi;
else
    y=u;
end

== matlab function PreCNN_SAC_RL_env/Inner Loop and Plant Model/High-FidelityModel with Autotuning/Plant Model/Bus setup/Generate GPS Data/Scale and Assemble GPS Data /Embedded MATLAB Function1 ==
  data: cog output; Vn input; Ve input
function cog = getCOG(Vn, Ve)
% This block supports an embeddable subset of the MATLAB language.
% See the help menu for details. 

cog = atan2(Ve,Vn);
if cog < 0;
    cog = cog + 2*pi;
end

== matlab function PreCNN_SAC_RL_env/Inner Loop and Plant Model/High-FidelityModel/MATLAB Function1 ==
  data: total_reward output; flags input; pos_curr input; pos_des input
function total_reward = Reward_Calculation(flags, pos_curr, pos_des)
    persistent min_reward_deviazione
    persistent max_reward_deviazione
    persistent max_deviazione
    persistent min_deviazione
    %persistent soglia_energia
    persistent deen_scaling
    persistent deviazione_scaling
    persistent penalty_crash
    persistent reward_goal
    persistent survival_bonus
    
    % inizializzazione costanti
    if isempty(min_deviazione)

        min_reward_deviazione = -1.0;
        max_reward_deviazione = 1.0;
        max_deviazione = 50.0;
        min_deviazione = 5.0;

        %soglia_energia = -200;

        deen_scaling = 1;
        deviazione_scaling = 1;

        penalty_crash = -500;
        reward_goal = 500;

        survival_bonus = 0.1;
    end
    
    % Inizializza il reward terminale a zero
    terminal_reward = 0;
    
    % Penalità collisione o schianto
    deviazione_eccessiva = flags(1);
    schianto_terra    = flags(2);
    collisione        = flags(3);
    
    if schianto_terra || collisione || deviazione_eccessiva
        terminal_reward = penalty_crash;
    end
    
    % Reward se raggiunge il goal
    traguardo_raggiunto = flags(4);
    
    if traguardo_raggiunto
        terminal_reward = reward_goal;
    end
    
    % Controllo deviazione
    % reward positivo da 0 a max se < min_deviazione,
    % reward negativo da 0 a min se > min_deviazione e < max_deviazione
    % deviazione: 0 min_deviazione/2 min_deviazione max_deviazione/2 max_deviazione
    % reward:     1        0.5             0               -0.5          -1
    deviazione_eccessiva = flags(1);
    reward_deviazione = min_reward_deviazione;
    if ~deviazione_eccessiva
        tracking_error = double(norm(pos_curr - pos_des));
        if tracking_error < min_deviazione
            reward_deviazione = max_reward_deviazione * (1.0 - tracking_error/min_deviazione);
        else
            reward_deviazione = min_reward_deviazione * tracking_error/max_deviazione;
        end
    end
    
    % Normalizzazione output DEEN per reward
    % alpha = -1;
    % reward_deen = alpha * (double(deen_output) - soglia_energia);
    % reward_deen = min(reward_deen, 500);
    % reward_deen = 1.0 - (1.0 / (1.0 + exp(reward_deen)));
    
    % total_reward = reward_deen * deen_scaling + terminal_reward ...
    %     + reward_deviazione * deviazione_scaling + survival_bonus;

    total_reward = terminal_reward ...
    + reward_deviazione * deviazione_scaling + survival_bonus;
    
end

== matlab function PreCNN_SAC_RL_env/Inner Loop and Plant Model/Low-FidelityModel/Assemble UAV State Bus/Generate GPS Data/Embedded MATLAB Function1 ==
  data: cog output; Vn input; Ve input
function cog = getCOG(Vn, Ve)
% This block supports an embeddable subset of the MATLAB language.
% See the help menu for details. 

cog = atan2(Ve,Vn);
if cog < 0;
    cog = cog + 2*pi;
end

== matlab function PreCNN_SAC_RL_env/Inner Loop and Plant Model/Low-FidelityModel/Position and Acceleration Control/Attitude Control/Multirotor Acceleration Control ==
  data: acc input; roll output; pitch output; yaw input; Gravity parameter
function [roll, pitch] = accControl(acc, yaw, Gravity)

    xddot = acc(1);
    yddot = acc(2);
    zddot = acc(3);
    
    pitch = atan2((-xddot*cos(yaw)-yddot*sin(yaw)), ( -zddot + Gravity));
    roll = atan2(((-xddot*sin(yaw)+yddot*cos(yaw))*cos(pitch)), (-zddot+Gravity));
    
end

== matlab function PreCNN_SAC_RL_env/Inner Loop and Plant Model/Low-FidelityModel/Position and Acceleration Control/Attitude Control/Multirotor Thrust Control ==
  data: acc input; pitch input; thrust output; roll input; DroneMass parameter; Gravity parameter
function thrust  = thrustControl(acc, pitch, roll, DroneMass, Gravity)

    zddot = acc(3);
    
    thrust = DroneMass*(-zddot+Gravity)/(cos(pitch)*cos(roll));
end

== matlab function PreCNN_SAC_RL_env/Inner Loop and Plant Model/High-FidelityModel/MATLAB Function2 ==
  data: flags input; isdone input; logging parameter; logPath_num parameter size=[1 250]; reward_curr input; t input
function logging_function(flags, isdone, logging, logPath_num, reward_curr, t)

    coder.extrinsic('fopen', 'fprintf', 'fclose');

    persistent total_steps
    persistent total_reward

    % --- GESTIONE VARIABILI PERSISTENTI E RESET ---
    if isempty(total_steps)
        total_steps = 0;
        total_reward = 0;
    end

    % Azzeramento sicuro: se t è 0, siamo all'inizio di un NUOVO episodio.
    % Azzeriamo i contatori qui per evitare bug se l'episodio precedente è andato in timeout.
    if t == 0
        total_steps = 0;
        total_reward = 0;
        return
    end

    % --- AGGIORNAMENTO STATISTICHE ---
    total_steps = total_steps + 1;
    total_reward = total_reward + reward_curr;

    % --- LOGGING ---
    if logging
        if isdone
            
            % Estrazione flag
            fuori_traiettoria = flags(1);
            schianto_terra    = flags(2);
            collisione        = flags(3);
            traguardo_raggiunto = flags(4);

            logPath = strtrim(char(logPath_num));
            fileID = -1;
            fileID = fopen(logPath, 'a'); 
            
            if fileID ~= -1
                if schianto_terra
                    fprintf(fileID, 'Step: %d | Rwd: %.2f | Motivo: Schianto a terra\n', int32(total_steps), double(total_reward));
                elseif collisione
                    fprintf(fileID, 'Step: %d | Rwd: %.2f | Motivo: Collisione ostacolo\n', int32(total_steps), double(total_reward));
                elseif fuori_traiettoria
                    fprintf(fileID, 'Step: %d | Rwd: %.2f | Motivo: Deviazione eccessiva\n', int32(total_steps), double(total_reward));
                elseif traguardo_raggiunto
                    fprintf(fileID, 'Step: %d | Rwd: %.2f | Motivo: TRAGUARDO RAGGIUNTO!\n', int32(total_steps), double(total_reward));
                end
                fclose(fileID);
            end
        end
    end
end

== matlab function PreCNN_SAC_RL_env/Inner Loop and Plant Model/High-FidelityModel/Control System/Controller/Position Controller/Position error transformation (Earth to Body frame) ==
  data: yaw input; xy_err_earth input; xy_err_body output
function xy_err_body = LTP2B2D(yaw,xy_err_earth)

transformation = [cos(yaw), sin(yaw); -sin(yaw),  cos(yaw)];
xy_err_body = transformation * xy_err_earth;


end

== matlab function PreCNN_SAC_RL_env/Inner Loop and Plant Model/High-FidelityModel/Control System/Controller/Position Controller/Velocity error transformation (Earth to Body frame) ==
  data: yaw input; xy_err_earth input; xy_err_body output
function xy_err_body = LTP2B2D(yaw,xy_err_earth)

transformation = [cos(yaw), sin(yaw); -sin(yaw),  cos(yaw)];
xy_err_body = transformation * xy_err_earth;


end

== matlab function PreCNN_SAC_RL_env/Inner Loop and Plant Model/High-FidelityModel/Control System/Controller/Yaw Controller/MATLAB Function ==
  data: u input; y output single
function y = wrapYaw(u)
%u error in rad in -2pi to 2pi

if (u>pi)
    y = single(u-2*pi);
elseif(u<-pi)
    y = single(u +2*pi);
else
    y=single(u);
end

== matlab function PreCNN_SAC_RL_env/Inner Loop and Plant Model/High-FidelityModel/Control System/Controller/Yaw Controller/MATLAB Function1 ==
  data: u input; y output
function y = wrapYaw(u)
%u error in rad in -2pi to 2pi

if (u>pi)
    y = u-2*pi;
elseif(u<-pi)
    y = u +2*pi;
else
    y=u;
end

== matlab function PreCNN_SAC_RL_env/Inner Loop and Plant Model/High-FidelityModel/Control System/Controller/Position Controller/Velocity error transformation (Earth to Body frame)1 ==
  data: yaw input; xy_err_earth input; xy_err_body output
function xy_err_body = LTP2B2D(yaw,xy_err_earth)

transformation = [cos(yaw), sin(yaw); -sin(yaw),  cos(yaw)];
xy_err_body = transformation * xy_err_earth;


end

== matlab function PreCNN_SAC_RL_env/Inner Loop and Plant Model/High-FidelityModel/State and Voxels extractor/MATLAB Function ==
  data: pos_drone input; voxel_flat output double; bounds parameter; t input; dyn_obs parameter
function voxel_flat = estrai_cubo_voxel(pos_drone, bounds, t, dyn_obs)
    res = 5.0; r = 5; margin = r * res;
    cubo = zeros(2*r, 2*r, 2*r, 'single');
    
    % 1. Estrazione cubo di voxel statico
    vicini_idx = find(~(bounds.x_max < pos_drone(1)-margin | bounds.x_min > pos_drone(1)+margin | ...
                        bounds.y_max < pos_drone(2)-margin | bounds.y_min > pos_drone(2)+margin | ...
                        bounds.z_max < pos_drone(3)-margin | bounds.z_min > pos_drone(3)+margin));
    
    % Creazione griglia 3D
    vx_range = pos_drone(1) - (r-0.5)*res : res : pos_drone(1) + (r-0.5)*res;
    vy_range = pos_drone(2) - (r-0.5)*res : res : pos_drone(2) + (r-0.5)*res;
    vz_range = pos_drone(3) - (r-0.5)*res : res : pos_drone(3) + (r-0.5)*res;

    [VX, VY, VZ] = ndgrid(vx_range, vy_range, vz_range);
                        
    if ~isempty(vicini_idx)
        for i = 1:length(vicini_idx)
            idx = vicini_idx(i);
            in_x = (VX >= bounds.x_min(idx)) & (VX <= bounds.x_max(idx));
            in_y = (VY >= bounds.y_min(idx)) & (VY <= bounds.y_max(idx));
            in_z = (VZ >= bounds.z_min(idx)) & (VZ <= bounds.z_max(idx));
            cubo(in_x & in_y & in_z) = 1;
        end
    end
    
    % 2. Sovrascrittura voxel se c'è un ostacolo dinamico nelle vicinanze
    for k = 1:length(dyn_obs)
        % Calcola la posizione attuale dell'ostacolo: P(t) = P0 + V*t
        pos_obs_corrente = dyn_obs(k).p0 + dyn_obs(k).v * t;
        
        % Controlla se la posizione dell'ostacolo è dentro il raggio 
        % d'azione del cubo locale del drone
        distanza_relativa = norm(pos_obs_corrente - pos_drone);
        
        if distanza_relativa < (margin + dyn_obs(k).radius)
            % Calcola la distanza al quadrato tra l'ostacolo e tutti i voxel della griglia
            dist_sq_grid = (VX - pos_obs_corrente(1)).^2 + (VY - pos_obs_corrente(2)).^2 + (VZ - pos_obs_corrente(3)).^2;
            
            % Tutti i voxel che ricadono dentro il raggio vengono messi a 1
            cubo(dist_sq_grid <= (dyn_obs(k).radius^2)) = 1;
        end
    end

    voxel_flat = cubo(:)';
    voxel_flat = double(voxel_flat);
end

== matlab function PreCNN_SAC_RL_env/Inner Loop and Plant Model/High-FidelityModel/Plant Model/Bus setup/Generate GPS Data/Scale and Assemble GPS Data /Embedded MATLAB Function1 ==
  data: cog output; Vn input; Ve input
function cog = getCOG(Vn, Ve)
% This block supports an embeddable subset of the MATLAB language.
% See the help menu for details. 

cog = atan2(Ve,Vn);
if cog < 0;
    cog = cog + 2*pi;
end

== matlab function PreCNN_SAC_RL_env/Inner Loop and Plant Model/High-FidelityModel with Autotuning/Control System/Controller/Position Controller/Position error transformation (Earth to Body frame) ==
  data: yaw input; xy_err_earth input; xy_err_body output
function xy_err_body = LTP2B2D(yaw,xy_err_earth)

transformation = [cos(yaw), sin(yaw); -sin(yaw),  cos(yaw)];
xy_err_body = transformation * xy_err_earth;


end

== matlab function PreCNN_SAC_RL_env/Inner Loop and Plant Model/High-FidelityModel/MATLAB Function ==
  data: tracking_error output; pos_curr input; isdone output; pos_des input; voxel_flat input; pos_goal parameter size=[1 3]; flags output; t input
function [tracking_error, isdone, flags] = check_terminal_state(pos_curr, pos_des, voxel_flat, pos_goal, t)

    persistent tolleranza_goal
    persistent max_deviazione

    if isempty(tolleranza_goal)
        tolleranza_goal = 1.0; % Raggio di accettazione

        max_deviazione = 100.0; % Limite di tolleranza deviazione in metri
    end

    pos_curr = pos_curr';
    pos_des = pos_des';


    % Ignora forzatamente il primo loop (t = 0)
    if t == 0
        isdone = false;
        flags = [false, false, false, false];
        distanza_goal = 0;
        tracking_error = 0;
        return; % Esce immediatamente dalla funzione
    end
    
    % 1. Controllo Divergenza (Tracking Error)
    % Calcola la distanza euclidea tra la posizione attuale e quella desiderata
    tracking_error = double(norm(pos_curr - pos_des));
    fuori_traiettoria = tracking_error > max_deviazione;
    
    % 2. Controllo Altitudine (Schianto a terra)
    % Presumendo che pos_curr(3) sia l'altitudine (asse Z positivo verso l'alto)
    quota_minima = 0;
    schianto_terra = pos_curr(3) < quota_minima;
    
    % 3. Controllo Collisione tramite Voxel
    % Rimodelliamo il vettore piatto nel cubo 10x10x10
    cubo = reshape(voxel_flat, [10, 10, 10]);
    
    % Controlliamo il "core" del drone (un nucleo di 2x2x2 voxel al centro)
    % Se almeno uno di questi voxel è 1, il drone ha colliso
    nucleo_centrale = cubo(5:6, 5:6, 5:6);
    collisione = any(nucleo_centrale == 1, 'all');

    % Controllo Traguardo Raggiunto
    distanza_goal = double(norm(pos_curr - pos_goal));
    traguardo_raggiunto = distanza_goal < tolleranza_goal;

    flags = [fuori_traiettoria, schianto_terra, collisione, traguardo_raggiunto];
    
    % L'episodio termina se si verifica ALMENO UNA di queste condizioni
    isdone = fuori_traiettoria | schianto_terra | collisione | traguardo_raggiunto;
    
end
